simulink model "setpoint_xd"  (R2017b)
settings: Solver=ode4  StartTime=0.0  StopTime=60  FixedStep=0.1  RelTol=1e-3
libraries: fuzblock x1
settings Model: Creator=phamt  LastModifiedBy=phamt

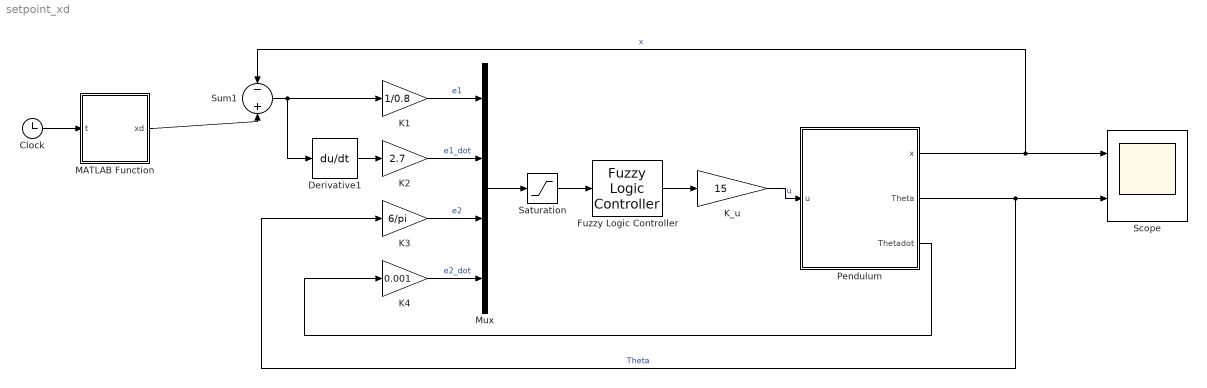
== system setpoint_xd ==
  Clock : Clock
      settings: Decimation=60
  Derivative1 : Derivative
  Fuzzy Logic Controller : fuzblock/Fuzzy Logic  Controller  FIS='bai2_FIS.fis'  OutputSampleNumber=101  DataType=double  FuzzifiedInputs=off  RuleFiringStrengths=off  RuleOutputs=off  AggregatedOutputs=off  SimulateUsing=Interpreted execution
  K1 : Gain  Gain=1/0.8
  K2 : Gain  Gain=2.7
  K3 : Gain  Gain=6/pi
  K4 : Gain  Gain=0.001
  K_u : Gain  Gain=15
  MATLAB Function : MATLAB Function  TreatAsAtomicUnit=on
  Mux : Mux
  Pendulum : Subsystem  mask{H=0.5, m=2, l=0.6, g=9.81, x0=0, xdot0=0, Theta0=0, Thetadot0=0.1}
      mask prompts: H "M"
  Saturation : Saturate  UpperLimit=1  LowerLimit=-1
  Scope : Scope  NumInputPorts=2
  Sum1 : Sum  Inputs=-+
  wires:
  Mux/1 -> Saturation/1
  K2/1 -> Mux/2  "e1_dot"
  K1/1 -> Mux/1  "e1"
  Fuzzy Logic Controller/1 -> K_u/1
  Saturation/1 -> Fuzzy Logic Controller/1
  K4/1 -> Mux/4  "e2_dot"
  K3/1 -> Mux/3  "e2"
  Derivative1/1 -> K2/1
  Clock/1 -> MATLAB Function/1(t)
  K_u/1 -> Pendulum/1(u)  "u"
  Sum1/1 -> Derivative1/1, K1/1
  MATLAB Function/1(xd) -> Sum1/2
  Pendulum/1(x) -> Sum1/1, Scope/1  "x"
  Pendulum/2(Theta) -> K3/1, Scope/2  "Theta"
  Pendulum/3(Thetadot) -> K4/1

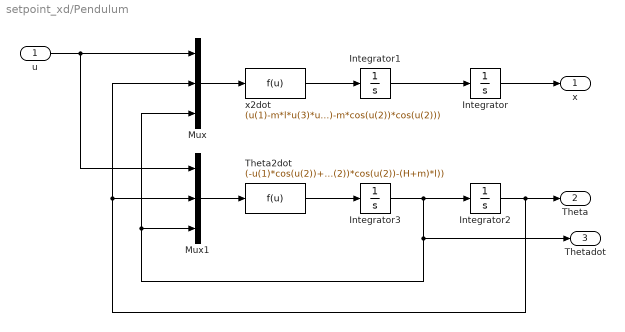
== system setpoint_xd/Pendulum ==
  u : Inport
  Integrator : Integrator  InitialCondition=x0
  Integrator1 : Integrator  InitialCondition=xdot0
  Integrator2 : Integrator  InitialCondition=Theta0
  Integrator3 : Integrator  InitialCondition=Thetadot0
  Mux : Mux  Inputs=3
  Mux1 : Mux  Inputs=3
  Theta2dot : Fcn  Expr=(-u(1)*cos(u(2))+m*g*u(3)*u(3)*sin(u(2))*cos(u(2))+(H+m)*(g*sin(u(2)))/(m*l*cos(u(2))*cos(u(2))-(H+m)*l))
  x2dot : Fcn  Expr=(u(1)-m*l*u(3)*u(3)*sin(u(2))-m*g*sin(u(2))*cos(u(2)))/((H+m)-m*cos(u(2))*cos(u(2)))
  x : Outport
  Theta : Outport  Port=2
  Thetadot : Outport  Port=3
  wires:
  x2dot/1 -> Integrator1/1
  Integrator/1 -> x/1
  Integrator1/1 -> Integrator/1
  Integrator3/1 -> Integrator2/1, Thetadot/1, Mux/3, Mux1/3
  Theta2dot/1 -> Integrator3/1
  u/1 -> Mux/1, Mux1/1
  Integrator2/1 -> Mux/2, Mux1/2, Theta/1
  Mux/1 -> x2dot/1
  Mux1/1 -> Theta2dot/1

== matlab function setpoint_xd/MATLAB Function ==
  data: t input; xd output
function xd = fcn(t)
if (0<=t) && (t<10)  
    xd = 0.45;
elseif (10<=t) &&(t<20) 
    xd = 0.2;
elseif (20<=t) &&(t<30)  
    xd = 0.8;
elseif (30<=t) &&(t<40)  
    xd = 0.55;
elseif (40<=t) &&(t<50)  
    xd = 0.1;
elseif (50<=t) &&(t<60)  
    xd = 0.65;
else xd = 0;
end
end
